simulink library "lib_new_data_verify"  (R2023b)
settings: Solver=VariableStepAuto  StartTime=0.0  StopTime=10.0  RelTol=1e-3
settings Model: Creator=Administrator  LastModifiedBy=bowen
settings SolverCC: AlgebraicLoopSolver=TrustRegion
settings DebuggingCC: UnconnectedInputMsg=warning  UnconnectedOutputMsg=warning  UnconnectedLineMsg=warning
settings ModelReferenceCC: EnableRefExpFcnMdlSchedulingChecks=on

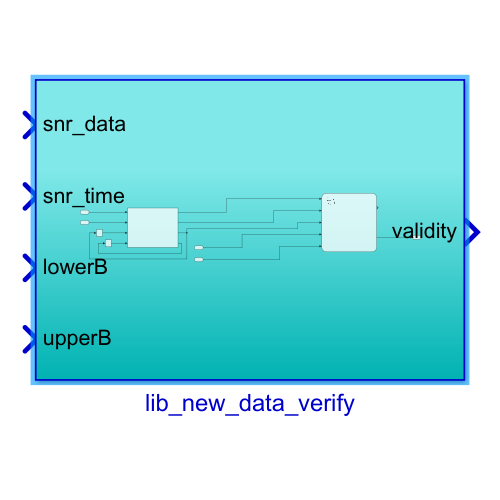
[thumbnail: Simulink's stored preview of the top-level diagram]
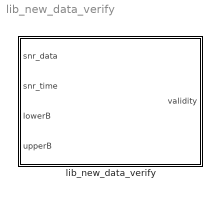
== system lib_new_data_verify ==
  lib_new_data_verify : Subsystem

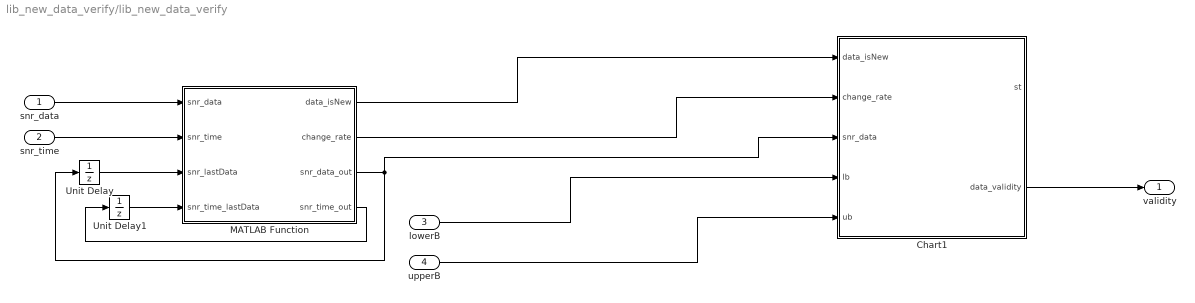
== system lib_new_data_verify/lib_new_data_verify ==
  snr_data : Inport  OutDataTypeStr=single
  snr_time : Inport  Port=2  OutDataTypeStr=single
  lowerB : Inport  Port=3  OutDataTypeStr=single
  upperB : Inport  Port=4  OutDataTypeStr=single
  Chart1 : Stateflow chart  TreatAsAtomicUnit=on
  MATLAB Function : MATLAB Function  TreatAsAtomicUnit=on
  Unit Delay : UnitDelay  SampleTime=-1  HasFrameUpgradeWarning=on
  Unit Delay1 : UnitDelay  SampleTime=-1  HasFrameUpgradeWarning=on
  validity : Outport
  wires:
  snr_time/1 -> MATLAB Function/2(snr_time)
  Unit Delay1/1 -> MATLAB Function/4(snr_time_lastData)
  Unit Delay/1 -> MATLAB Function/3(snr_lastData)
  MATLAB Function/1(data_isNew) -> Chart1/1(data_isNew)
  snr_data/1 -> MATLAB Function/1(snr_data)
  MATLAB Function/4(snr_time_out) -> Unit Delay1/1
  lowerB/1 -> Chart1/4(lb)
  upperB/1 -> Chart1/5(ub)
  MATLAB Function/2(change_rate) -> Chart1/2(change_rate)
  MATLAB Function/3(snr_data_out) -> Unit Delay/1, Chart1/3(snr_data)
  Chart1/2(data_validity) -> validity/1

== stateflow chart lib_new_data_verify/Chart1 ==
  state No
    en:
    st = 0;
    data_validity = false;
  state possible1
    en:
    st = 1;
  state comfirmed
    en:
    st = 2;
  state done
    en:
    st = 3;
    data_validity = true;
  (default) -> No
  possible1 -> No [order 3] : after(0.01, sec)
  possible1 -> No [order 1] : [    ( data > ub ) ...
      |   || ( data < lb ) ]
  No -> (junction 6) : [data_isNew]
  (junction 6) -> possible1 : [    ( snr_data < ub) ...
      | && ( snr_data > lb) ]
  possible1 -> (junction 13) [order 2] : [data_isNew]
  (junction 13) -> comfirmed : [   ( snr_data < ub) ...
      | && ( snr_data > lb) ]
  comfirmed -> done : after(0.01, sec)
  data: data_isNew input boolean; change_rate input double; snr_data input double; lb input double; ub input double; st output double; data_validity output boolean

== matlab function lib_new_data_verify/MATLAB Function ==
  data: snr_data input single; snr_time input single; data_isNew output boolean; change_rate output; snr_lastData input single; snr_time_lastData input single; snr_data_out output single; snr_time_out output single
function [data_isNew, change_rate, snr_data_out, snr_time_out] = fcn(snr_data, snr_time, snr_lastData, snr_time_lastData)

data_isNew = false; 
snr_data_out = snr_lastData;
snr_time_out = snr_time_lastData;
change_rate = single(0);


if ( snr_time - snr_time_lastData )> 0.001     % sec
    data_isNew = true;   
    change_rate = (snr_data - snr_lastData) / (snr_time - snr_time_lastData);
    snr_data_out = snr_data;
    snr_time_out = snr_time;
end
